simulink model "test_helper_smib"  (R2025b)
settings: Solver=FixedStepAuto  StartTime=0.0  StopTime=5  FixedStep=50e-6  RelTol=1e-3
undefined symbols (not defined in the file or in its folder): D_es1_test, delta0_es1_test, LoadStep_t_s, M_es1_test, Pe_scale, Pm_es1_test, Pm_step_amp_es1_test, Pm_step_t_es1_test, Vmag_es1_test, VSGScale_es1_test, wn_const
libraries: spsControlledVoltageSourceLib x3, spsSeriesRLCBranchLib x3, spsThreePhaseSeriesRLCLoadLib x2, spsThreePhaseBreakerLib x1, spsGroundLib x1, spsThreePhaseVIMeasurementLib x1, spspowerguiLib x1
settings Model: Creator=27443  LastModifiedBy=27443

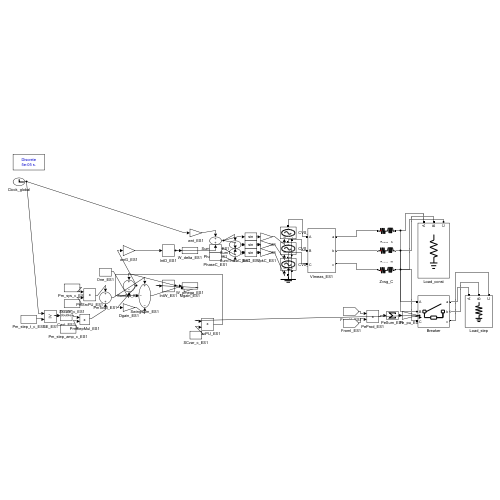
[thumbnail: Simulink's stored preview of the top-level diagram]
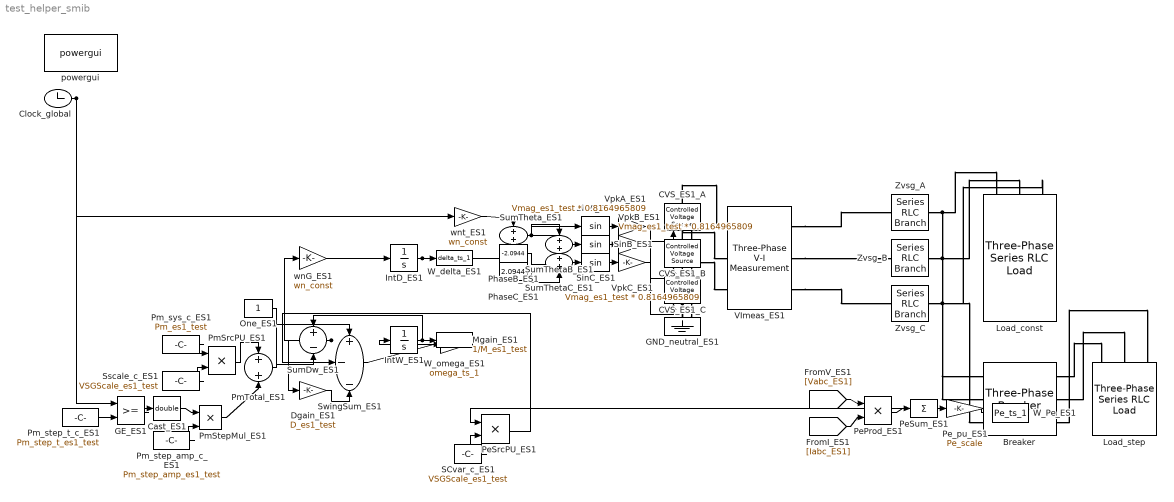
== system test_helper_smib ==
  Breaker : spsThreePhaseBreakerLib/Three-Phase Breaker  InitialState=open  SwitchA=on  SwitchB=on  SwitchC=on  SwitchTimes=[LoadStep_t_s]  External=off  BreakerResistance=0.01  SnubberResistance=1e6  SnubberCapacitance=inf  Measurements=None
  CVS_ES1_A : spsControlledVoltageSourceLib/Controlled Voltage Source  Initialize=on  Source_Type=AC  Amplitude=0  Phase=0  Frequency=0  Measurements=None
  CVS_ES1_B : spsControlledVoltageSourceLib/Controlled Voltage Source  Initialize=on  Source_Type=AC  Amplitude=0  Phase=0  Frequency=0  Measurements=None
  CVS_ES1_C : spsControlledVoltageSourceLib/Controlled Voltage Source  Initialize=on  Source_Type=AC  Amplitude=0  Phase=0  Frequency=0  Measurements=None
  Cast_ES1 : DataTypeConversion  OutDataTypeStr=double  SaturateOnIntegerOverflow=off  RndMeth=Floor
  Clock_global : Clock
  Dgain_ES1 : Gain  Gain=D_es1_test
  GE_ES1 : RelationalOperator  OutDataTypeStr=boolean  RndMeth=Simplest  InputSameDT=off
  GND_neutral_ES1 : spsGroundLib/Ground  LConnTagsString=a
  IntD_ES1 : Integrator  InitialCondition=delta0_es1_test
  IntW_ES1 : Integrator  InitialCondition=1
  Load_const : spsThreePhaseSeriesRLCLoadLib/Three-Phase Series RLC Load  LConnTagsString=A|B|C  Configuration=Y (grounded)  NominalVoltage=230000  Vabc=[1e3 1e3 1e3]  Vabcp=[1e3 1e3 1e3]  NominalFrequency=50  UnbalancedPower=off  ActivePower=40e6  InductivePower=0  CapacitivePower=0  Pabc=[10e3 9e3 11e3]  QLabc=[100 90 110]  QCabc=[100 90 110]  Pabcp=[10e3 9e3 11e3]  QLabcp=[100 90 110]  QCabcp=[100 90 110]  Measurements=None  LoadType=constant Z
  Load_step : spsThreePhaseSeriesRLCLoadLib/Three-Phase Series RLC Load  LConnTagsString=A|B|C  Configuration=Y (grounded)  NominalVoltage=230000  Vabc=[1e3 1e3 1e3]  Vabcp=[1e3 1e3 1e3]  NominalFrequency=50  UnbalancedPower=off  ActivePower=LoadStep_amp_W  InductivePower=0  CapacitivePower=0  Pabc=[10e3 9e3 11e3]  QLabc=[100 90 110]  QCabc=[100 90 110]  Pabcp=[10e3 9e3 11e3]  QLabcp=[100 90 110]  QCabcp=[100 90 110]  Measurements=None  LoadType=constant Z
  Mgain_ES1 : Gain  Gain=1/M_es1_test
  One_ES1 : Constant
  PeProd_ES1 : Product
  PeSrcPU_ES1 : Product
  PeSum_ES1 : Sum  Inputs=+
  Pe_pu_ES1 : Gain  Gain=Pe_scale
  PhaseB_ES1 : Constant  Value=-2.0944
  PhaseC_ES1 : Constant  Value=2.0944
  PmSrcPU_ES1 : Product
  PmStepMul_ES1 : Product
  PmTotal_ES1 : Sum
  Pm_step_amp_c_ES1 : Constant  Value=Pm_step_amp_es1_test
  Pm_step_t_c_ES1 : Constant  Value=Pm_step_t_es1_test
  Pm_sys_c_ES1 : Constant  Value=Pm_es1_test
  SCvar_c_ES1 : Constant  Value=VSGScale_es1_test
  SinA_ES1 : Trigonometry
  SinB_ES1 : Trigonometry
  SinC_ES1 : Trigonometry
  Sscale_c_ES1 : Constant  Value=VSGScale_es1_test
  SumDw_ES1 : Sum  Inputs=+-
  SumThetaB_ES1 : Sum
  SumThetaC_ES1 : Sum
  SumTheta_ES1 : Sum
  SwingSum_ES1 : Sum  Inputs=+--
  VImeas_ES1 : spsThreePhaseVIMeasurementLib/Three-Phase V-I Measurement  VoltageMeasurement=phase-to-ground  SetLabelV=on  LabelV=Vabc_ES1  Vpu=off  VpuLL=off  CurrentMeasurement=yes  SetLabelI=on  LabelI=Iabc_ES1  Ipu=off  Pbase=100e6  Vbase=500e3  OutputType=Complex  PhasorSimulation=off  PSBequivalent=0
  VpkA_ES1 : Gain  Gain=Vmag_es1_test * 0.8164965809
  VpkB_ES1 : Gain  Gain=Vmag_es1_test * 0.8164965809
  VpkC_ES1 : Gain  Gain=Vmag_es1_test * 0.8164965809
  W_Pe_ES1 : ToWorkspace  VariableName=Pe_ts_1  SaveFormat=Timeseries  SampleTime=-1
      settings: MaxDataPoints=2
  W_delta_ES1 : ToWorkspace  VariableName=delta_ts_1  SaveFormat=Timeseries  SampleTime=-1
      settings: MaxDataPoints=2
  W_omega_ES1 : ToWorkspace  VariableName=omega_ts_1  SaveFormat=Timeseries  SampleTime=-1
      settings: MaxDataPoints=2
  Zvsg_A : spsSeriesRLCBranchLib/Series RLC Branch  LConnTagsString=__new0  RConnTagsString=__new0  BranchType=RL  Resistance=0.7935  Inductance=0.25258  SetiL0=off  InitialCurrent=0  Capacitance=1e-6  Setx0=off  InitialVoltage=0  Measurements=None
  Zvsg_B : spsSeriesRLCBranchLib/Series RLC Branch  LConnTagsString=__new0  RConnTagsString=__new0  BranchType=RL  Resistance=0.7935  Inductance=0.25258  SetiL0=off  InitialCurrent=0  Capacitance=1e-6  Setx0=off  InitialVoltage=0  Measurements=None
  Zvsg_C : spsSeriesRLCBranchLib/Series RLC Branch  LConnTagsString=__new0  RConnTagsString=__new0  BranchType=RL  Resistance=0.7935  Inductance=0.25258  SetiL0=off  InitialCurrent=0  Capacitance=1e-6  Setx0=off  InitialVoltage=0  Measurements=None
  powergui : spspowerguiLib/powergui  Priority=1  SimulationMode=Discrete  SampleTime=50e-6  frequency=60  Iterations=50  frequencyindice=60  Pbase=100e6  ErrMax=1e-4  UnitsV=kV  UnitsW=MW  buscounter=0  FunctionMessages=off  echomessages=off  EnableUseOfTLC=off  CurrentSourceSwitches=off  DisableSnubberDevices=off  DisableRonSwitches=off  DisableVfSwitches=off  DisplayEquations=off  AutomaticDiscreteSolvers=off  SolverType=Tustin/Backward Euler (TBE)  Interpol=off  ExternalGateDelay=off  methode=off  Ts=100  x0status=blocks  SPID=on  SwTol=0  HookPort=off  NonlinearTolerance=1e-4  nMaxIteration=100  ContinueOnMaxIteration=off  RestoreLinks=warning  ResistiveCurrentMeasurement=off  Frange=[0:2:500]  Ylog=off  Xlog=on  ShowGrid=off  save=off  variable=ZData  structure=0  ZoomFFT=off  StartTime=0.0  cycles=1  DisplayStyle=1  fundamental=60  FreqAxis=off  MaxFrequency=1000  frequencyindicesteady=1  RmsSteady=1  display=off
  wnG_ES1 : Gain  Gain=wn_const
  wnt_ES1 : Gain  Gain=wn_const
  wires:
  Clock_global/1 -> GE_ES1/1, wnt_ES1/1
  Pm_step_t_c_ES1/1 -> GE_ES1/2
  GE_ES1/1 -> Cast_ES1/1
  Cast_ES1/1 -> PmStepMul_ES1/1
  Pm_step_amp_c_ES1/1 -> PmStepMul_ES1/2
  Pm_sys_c_ES1/1 -> PmSrcPU_ES1/1
  Sscale_c_ES1/1 -> PmSrcPU_ES1/2
  PmSrcPU_ES1/1 -> PmTotal_ES1/1
  PmStepMul_ES1/1 -> PmTotal_ES1/2
  IntW_ES1/1 -> SumDw_ES1/1, W_omega_ES1/1
  One_ES1/1 -> SumDw_ES1/2
  SumDw_ES1/1 -> Dgain_ES1/1, wnG_ES1/1
  PmTotal_ES1/1 -> SwingSum_ES1/1
  Dgain_ES1/1 -> SwingSum_ES1/3
  SwingSum_ES1/1 -> Mgain_ES1/1
  Mgain_ES1/1 -> IntW_ES1/1
  wnG_ES1/1 -> IntD_ES1/1
  wnt_ES1/1 -> SumTheta_ES1/1
  IntD_ES1/1 -> SumTheta_ES1/2, W_delta_ES1/1
  SumTheta_ES1/1 -> SumThetaB_ES1/1, SumThetaC_ES1/1, SinA_ES1/1
  PhaseB_ES1/1 -> SumThetaB_ES1/2
  PhaseC_ES1/1 -> SumThetaC_ES1/2
  SumThetaB_ES1/1 -> SinB_ES1/1
  SumThetaC_ES1/1 -> SinC_ES1/1
  SinA_ES1/1 -> VpkA_ES1/1
  SinB_ES1/1 -> VpkB_ES1/1
  SinC_ES1/1 -> VpkC_ES1/1
  VpkA_ES1/1 -> CVS_ES1_A/1
  VpkB_ES1/1 -> CVS_ES1_B/1
  VpkC_ES1/1 -> CVS_ES1_C/1
  [Vabc_ES1] -> PeProd_ES1/1
  [Iabc_ES1] -> PeProd_ES1/2
  PeProd_ES1/1 -> PeSum_ES1/1
  PeSum_ES1/1 -> Pe_pu_ES1/1
  Pe_pu_ES1/1 -> PeSrcPU_ES1/1, W_Pe_ES1/1
  SCvar_c_ES1/1 -> PeSrcPU_ES1/2
  PeSrcPU_ES1/1 -> SwingSum_ES1/2
  connections:
  CVS_ES1_A/LConn1 -- CVS_ES1_B/LConn1 -- GND_neutral_ES1/LConn1 -- CVS_ES1_C/LConn1
  CVS_ES1_A/RConn1 -- VImeas_ES1/LConn1
  CVS_ES1_B/RConn1 -- VImeas_ES1/LConn2
  CVS_ES1_C/RConn1 -- VImeas_ES1/LConn3
  VImeas_ES1/RConn1 -- Zvsg_A/LConn1
  VImeas_ES1/RConn2 -- Zvsg_B/LConn1
  VImeas_ES1/RConn3 -- Zvsg_C/LConn1
  Load_const/LConn1 -- Zvsg_A/RConn1 -- Breaker/LConn1
  Load_const/LConn2 -- Zvsg_B/RConn1 -- Breaker/LConn2
  Load_const/LConn3 -- Zvsg_C/RConn1 -- Breaker/LConn3
  Breaker/RConn1 -- Load_step/LConn1
  Breaker/RConn2 -- Load_step/LConn2
  Breaker/RConn3 -- Load_step/LConn3
